simulink model "QPSK_ad9361_Solution"  (R2019a)
settings: Solver=ode23  StartTime=0.0  StopTime=inf  RelTol=1e-3  EnableMultiTasking=on
PreLoadFcn:
  | addpath('./filterwizard');
  | ad9361_preload(bdroot,'rx');
  | sdrqpsktx = qpsktx_init;
  | sdrqpskrx = qpskrx_init;
InitFcn:
  | sdrqpsktx = qpsktx_init;
  | sdrqpskrx = qpskrx_init;
undefined symbols (not defined in the file or in its folder): D, dBc, dBval, DCLeak_Matrix, dfilt, doppler, errordlg, Frame, fuzz_val, GainImb_Matrix, gcbh, IP2_Matrix, IP3_Matrix, magnitude, rcfiltgaincompat
libraries: simrfV2elements x23, dspmlti4 x10, simrfV2util1 x9, simulink x9, dsparch4 x8, fl_lib x7, dspmathops x5, dspobslib x4, simrfV2sources1 x3, simrfV2junction1 x3, commdigbbndpm3 x3, dspstat3 x3
(part 3 of 3)

== system QPSK_ad9361_Solution/ADI9361_tx1/DUC_Filters_TX/Hm3/Hm3 ==
  In : Inport
  Hm3 : dspmlti4/FIR Interpolation  FilterSource=Filter object  h=fir1(15,1/4)  L=3  FilterObject=ad9361_tx_pars.Hm3_tx  framing=Allow multirate processing  outputBufInitCond=0  roundingMode=Floor  overflowMode=off  firstCoeffDataTypeStr=Inherit: Same word length as input  firstCoeffMin=[]  firstCoeffMax=[]  firstCoeffLastDataTypeStr=Inherit: Same word length as input  outputDataTypeStr=Inherit: Same as accumulator  outputMin=[]  outputMax=[]  outputLastDataTypeStr=Inherit: Same as accumulator
      settings: SourceProductName=DSP System Toolbox
  Out : Outport
  wires:
  Hm3/1 -> Out/1
  In/1 -> Hm3/1

== system QPSK_ad9361_Solution/ADI9361_tx1/DUC_Filters_TX/Hm3/NoFilter ==
  In : Inport
  Out : Outport
  wires:
  In/1 -> Out/1

== system QPSK_ad9361_Solution/ADI9361_tx1/DUC_Filters_TX/Hm4/Hm4 ==
  In1 : Inport
  Hm4 : dspmlti4/FIR Interpolation  FilterSource=Filter object  h=fir1(15,1/4)  L=3  FilterObject=ad9361_tx_pars.Hm4_tx  framing=Allow multirate processing  outputBufInitCond=0  roundingMode=Floor  overflowMode=off  firstCoeffDataTypeStr=Inherit: Same word length as input  firstCoeffMin=[]  firstCoeffMax=[]  firstCoeffLastDataTypeStr=Inherit: Same word length as input  outputDataTypeStr=Inherit: Same as accumulator  outputMin=[]  outputMax=[]  outputLastDataTypeStr=Inherit: Same as accumulator
      settings: SourceProductName=DSP System Toolbox
  Out1 : Outport
  wires:
  Hm4/1 -> Out1/1
  In1/1 -> Hm4/1

== system QPSK_ad9361_Solution/ADI9361_tx1/DUC_Filters_TX/Hm4/NoFilter ==
  In1 : Inport
  Out1 : Outport
  wires:
  In1/1 -> Out1/1

== system QPSK_ad9361_Solution/ADI9361_tx1/RF_TX/Modulator/Combiner ==
  Gnd : fl_lib/Electrical/Electrical Elements/Electrical Reference
  Rl_I : simrfV2elements/R  classname=resistor  Resistance=50 Ohm  AddNoise=off
      settings: SourceProductName=RF Blockset  SourceProductBaseCode=RB
  Rl_Q : simrfV2elements/R  classname=resistor  Resistance=50 Ohm  AddNoise=off
      settings: SourceProductName=RF Blockset  SourceProductBaseCode=RB
  Rs : simrfV2elements/R  classname=resistor  Resistance=50 Ohm  AddNoise=off
      settings: SourceProductName=RF Blockset  SourceProductBaseCode=RB
  Signal Combiner : simrfV2elements/Signal Combiner  classname=signal_sum_mask  InternalGrounding=on
      settings: SourceProductName=RF Blockset  SourceProductBaseCode=RB
  In1 : PMIOPort  Side=Left
  In2 : PMIOPort  Port=2  Side=Left
  Out : PMIOPort  Port=3  Side=Right
  connections:
  Rs/RConn1 -- Signal Combiner/RConn1
  Rs/LConn1 -- Out/RConn1
  Rl_I/LConn1 -- In1/RConn1 -- Signal Combiner/LConn1
  Rl_Q/RConn1 -- In2/RConn1 -- Signal Combiner/LConn2
  Rl_I/RConn1 -- Rl_Q/LConn1 -- Gnd/LConn1

== system QPSK_ad9361_Solution/ADI9361_tx1/RF_TX/Modulator/GainImbalance = f(Attenuation,Imp) ==
  Attenuation : Inport
  1-D Lookup Table : Lookup_n-D  NumberOfTableDimensions=1  BreakpointsForDimension1="[    0    10    20    30    40    50    60    70    80]"  BreakpointsForDimension1FirstPoint=10  BreakpointsForDimension2FirstPoint=10  BreakpointsForDimension1Spacing=12  BreakpointsForDimension2Spacing=12  Table="[-55.5 -66.2 -53.5 -57.5 -44.5 -46.3 -54.2 -46.1 -34.3] / 20     %[dBc]"  InternalRulePriority=Speed  RndMeth=Simplest  InputSameDT=on
  Add : Sum
  Constant : Constant
  Control : Constant  Value=Imp
  Gain : Gain  Gain=20
  Gain1 : Gain  Gain=2
  Power : Math  Operator=10^u  SaturateOnIntegerOverflow=on
  Switch : Switch  Criteria=u2 ~= 0
  Zero : Constant  Value=0
  log10 : Math  Operator=log10  SaturateOnIntegerOverflow=on
  GainImbalance : Outport
  wires:
  log10/1 -> Gain/1
  Attenuation/1 -> 1-D Lookup Table/1
  Zero/1 -> Switch/3
  1-D Lookup Table/1 -> Power/1
  Gain/1 -> Switch/1
  Constant/1 -> Add/2
  Control/1 -> Switch/2
  Power/1 -> Gain1/1
  Gain1/1 -> Add/1
  Add/1 -> log10/1
  Switch/1 -> GainImbalance/1

== system QPSK_ad9361_Solution/ADI9361_tx1/RF_TX/Modulator/Noisy LO ==
  Constant : Constant  Value=sqrt(2)  VectorParams1D=off  SampleTime=1/Fs  FramePeriod=Frame/Fs
  Phase Noise : Subsystem  Description=|  mask{Level_dB=Level_dB, Freq=Freq, Fs=Fs, Npts=Npts, seed=seed, Verify=off}
      | User defined phase noise block.
      | Dick Benson, May 2007
      mask prompts: Level_dB "Noise Level Vector in dBc/Hz"; Freq "Frequency Vector in Hz"; Fs "Sampling Rate in Hz"; Npts "FIR Filter Kernel Length (power of 2)"; seed "Noise Gen. Seed"; Verify "Verify Noise Shape Attained"
      mask init:
      | noise_filt = phasenoise(Npts, Freq, Level_dB, Fs, Verify, gcb);
      mask Display: disp('Prototype\nPhase Noise\nBlock')
  Real-Imag to Complex : RealImagToComplex  Input=Real
  PLL Output : Outport
  wires:
  Constant/1 -> Real-Imag to Complex/1
  Real-Imag to Complex/1 -> Phase Noise/1(In1)
  Phase Noise/1(Out1) -> PLL Output/1

== system QPSK_ad9361_Solution/ADI9361_tx1/RF_TX/Modulator/R = f(Attenuation,Gain,Imp) ==
  Attenuation : Inport
  Add : Sum  Inputs=+-
  Constant : Constant  Value=50
  Constant2 : Constant  Value=1e21
  Control : Constant  Value=Imp
  Gain : Gain  Gain=50*50
  Lookup Table : Lookup_n-D  NumberOfTableDimensions=1  BreakpointsForDimension1="[  0  10  20  30  40  50   60   70   80]"  BreakpointsForDimension1FirstPoint=10  BreakpointsForDimension2FirstPoint=10  BreakpointsForDimension1Spacing=12  BreakpointsForDimension2Spacing=12  Table=-1*([-58 -52 -60 -71 -81 -82 -101 -102 -100] - Gain - 6)/10  InternalRulePriority=Speed  RndMeth=Simplest  InputSameDT=on
  Sqrt : Sqrt  SaturateOnIntegerOverflow=on
  Switch : Switch  Criteria=u2 ~= 0
  expon : Math  Operator=10^u  SaturateOnIntegerOverflow=on
  R : Outport
  wires:
  Constant/1 -> Add/2
  Lookup Table/1 -> expon/1
  Attenuation/1 -> Lookup Table/1
  Sqrt/1 -> Add/1
  Gain/1 -> Sqrt/1
  Control/1 -> Switch/2
  Switch/1 -> R/1
  Constant2/1 -> Switch/3
  Add/1 -> Switch/1
  expon/1 -> Gain/1

== system QPSK_ad9361_Solution/ADI9361_tx1/RF_TX/PA/OIP3 = f(Attenuation,OIP3v,Imp) ==
  Attenuation : Inport
  1-D Lookup Table : Lookup_n-D  NumberOfTableDimensions=1  BreakpointsForDimension1=[0 4 20 80]  BreakpointsForDimension1FirstPoint=10  BreakpointsForDimension2FirstPoint=10  BreakpointsForDimension1Spacing=12  BreakpointsForDimension2Spacing=12  Table=OIP3v  InternalRulePriority=Speed  RndMeth=Simplest  InputSameDT=on
  Constant2 : Constant  Value=500
  Control : Constant  Value=Imp
  Switch : Switch  Criteria=u2 ~= 0
  OIP3 : Outport
  wires:
  1-D Lookup Table/1 -> Switch/1
  Attenuation/1 -> 1-D Lookup Table/1
  Control/1 -> Switch/2
  Switch/1 -> OIP3/1
  Constant2/1 -> Switch/3

== system QPSK_ad9361_Solution/QPSK Receiver/Timing Recovery1/Modified Buffer/Modified Buffer ==
  In1 : Inport
  Enable : EnablePort
  Compare To Constant : simulink/Logic and Bit Operations/Compare To Constant  relop===  const=(bufSize-1)  OutDataTypeStr=boolean  ZeroCross=off
  Counter Limited : simulink/Sources/Counter Limited  uplimit=(bufSize-1)  tsamp=-1
  Delay Line : dspbuff3/Delay Line  siz=bufSize  ic=0  directfeed=on  enable_output=on  hold_output=off  OutputFrames=on
      settings: SourceProductName=DSP System Toolbox  SourceProductBaseCode=DS
  DataOut : Outport
  DataValid : Outport  Port=2
  wires:
  Compare To Constant/1 -> Delay Line/2, DataValid/1
  Delay Line/1 -> DataOut/1
  In1/1 -> Delay Line/1
  Counter Limited/1 -> Compare To Constant/1

== system QPSK_ad9361_Solution/QPSK Receiver/Timing Recovery1/Timing Recovery PLL/Loop Filter ==
  note: Proportional-Plus-Integrator Loop Filter,
      | Infinite DC Response to guarantee convergence
  e : Inport
  Digital Filter : dspobslib/Digital Filter  TypePopup=IIR (poles & zeros)  IIRFiltStruct=Direct form II transposed  AllPoleFiltStruct=Direct form  FIRFiltStruct=Direct form  CoeffSource=Specify via dialog  NumCoeffs=[1 0]  DenCoeffs=[1 -1]  BiQuadCoeffs=[1 0.3 0.4 1 0.1 0.2]  LatticeCoeffs=[0.2 0.4]  denIgnore=on  FiltPerSampPopup=One filter per frame  IC=0  ICnum=0  ICden=0  roundingMode=Floor  overflowMode=off  ScaleValues=1  scaleValueFracLength=14  stageInFracLength=15  stageOutFracLength=15  FilterSource=Specify via dialog  dfiltObjectName=dfilt.dffir([1 2 1])  InputProcessing=Columns as channels (frame based)
      settings: SourceProductName=DSP System Toolbox  SourceProductBaseCode=DS
  K1 : Gain  Gain=K1
  K2 : Gain  Gain=K2
  Sum2 : Sum  SaturateOnIntegerOverflow=on  InputSameDT=on  OutDataTypeStr=Inherit: Same as first input
  v : Outport
  wires:
  K2/1 -> Digital Filter/1
  Digital Filter/1 -> Sum2/2
  Sum2/1 -> v/1
  e/1 -> K2/1, K1/1
  K1/1 -> Sum2/1

== system QPSK_ad9361_Solution/ADI9361_rx1/RF_RX/RF Receiver/Demodulator/R = f(gain, DCleak) ==
  gain : Inport
  DCleak : Inport  Port=2
  Add : Sum  Inputs=--+-+
  Add1 : Sum  Inputs=+-
  Constant1 : Constant  Value=20
  Constant2 : Constant  Value=27
  Constant3 : Constant  Value=3
  Constant4 : Constant  Value=25
  Gain1 : Gain  Gain=(-1)/20
  Gain2 : Gain  Gain=25
  expon3 : Math  Operator=10^u  SaturateOnIntegerOverflow=on
  R : Outport
  wires:
  Add1/1 -> R/1
  Constant4/1 -> Add1/2
  Gain2/1 -> Add1/1
  Gain1/1 -> expon3/1
  Constant2/1 -> Add/4
  Constant1/1 -> Add/3
  Constant3/1 -> Add/2
  DCleak/1 -> Add/5
  Add/1 -> Gain1/1
  gain/1 -> Add/1
  expon3/1 -> Gain2/1

== system QPSK_ad9361_Solution/ADI9361_rx1/RF_RX/RF Receiver/Demodulator/y = f(gain, gainImbalance) ==
  gain : Inport
  gainImbalance : Inport  Port=2
  Add2 : Sum
  Constant2 : Constant  Value=2
  Gain4 : Gain  Gain=1/20
  Gain5 : Gain  Gain=1/20
  Gain6 : Gain  Gain=20
  Times1 : Product  Inputs=***
  expon2 : Math  Operator=10^u  SaturateOnIntegerOverflow=on
  expon3 : Math  Operator=10^u  SaturateOnIntegerOverflow=on
  log1 : Math  Operator=log10  SaturateOnIntegerOverflow=on
  y : Outport
  wires:
  expon2/1 -> Times1/2
  Gain5/1 -> expon3/1
  Times1/1 -> Add2/2
  Gain4/1 -> expon2/1
  Add2/1 -> log1/1
  log1/1 -> Gain6/1
  gain/1 -> Gain5/1
  expon3/1 -> Times1/1, Add2/1
  gainImbalance/1 -> Gain4/1
  Constant2/1 -> Times1/3
  Gain6/1 -> y/1

== system QPSK_ad9361_Solution/ADI9361_rx1/RF_RX/RF Receiver/External LNA/Invert Control ==
  In : Inport
  Data Type Conversion : DataTypeConversion  OutDataTypeStr=boolean
  Data Type Conversion1 : DataTypeConversion  OutDataTypeStr=double
  Logical Operator : Logic  Operator=NOT  AllPortsSameDT=off  OutDataTypeStr=boolean
  Out : Outport
  wires:
  In/1 -> Data Type Conversion/1
  Logical Operator/1 -> Data Type Conversion1/1
  Data Type Conversion/1 -> Logical Operator/1
  Data Type Conversion1/1 -> Out/1

== system QPSK_ad9361_Solution/ADI9361_rx1/RF_RX/RF Receiver/RF Non Idealities/DetectChange ==
  In1 : Inport
  In2 : Inport  Port=2
  In3 : Inport  Port=3
  In4 : Inport  Port=4
  Detect Change{,1..4} (5 alike) : simulink/Logic and Bit Operations/Detect Change  vinit=0  InputProcessing=Inherited  OutDataTypeStr=boolean
  Logical Operator : Logic  Operator=OR  Inputs=5  AllPortsSameDT=off  OutDataTypeStr=boolean
  Step : Step  Time=2*Tstep  SampleTime=Tstep  VectorParams1D=off  ZeroCross=off
  Trigger : Outport
  wires:
  Detect Change/1 -> Logical Operator/4
  Detect Change1/1 -> Logical Operator/3
  Detect Change2/1 -> Logical Operator/2
  In4/1 -> Detect Change3/1
  In2/1 -> Detect Change1/1
  In3/1 -> Detect Change2/1
  Detect Change3/1 -> Logical Operator/1
  In1/1 -> Detect Change/1
  Logical Operator/1 -> Trigger/1
  Detect Change4/1 -> Logical Operator/5
  Step/1 -> Detect Change4/1

== system QPSK_ad9361_Solution/ADI9361_rx1/RF_RX/RF Receiver/RF Non Idealities/RF Non Idealities ==
  LNA : Inport
  Demod : Inport  Port=2
  TIA : Inport  Port=3
  LPF : Inport  Port=4
  Trigger : TriggerPort  VariantControl=Variant  PortDimensions=1
  RF NonIdealities : MATLAB Function  TreatAsAtomicUnit=on
      mask init:
      | load ADI9361Tables;
  DCLeakage : Outport
  GainImbalance : Outport  Port=2
  IP2 : Outport  Port=3
  IP3 : Outport  Port=4
  wires:
  RF NonIdealities/1(Leak) -> DCLeakage/1
  RF NonIdealities/2(GainImb) -> GainImbalance/1
  RF NonIdealities/3(IP2) -> IP2/1
  RF NonIdealities/4(IP3) -> IP3/1
  LNA/1 -> RF NonIdealities/1(LNA)
  LPF/1 -> RF NonIdealities/4(LPF)
  Demod/1 -> RF NonIdealities/2(Demod)
  TIA/1 -> RF NonIdealities/3(TIA)

== system QPSK_ad9361_Solution/ADI9361_tx1/RF_TX/Modulator/Noisy LO/Phase Noise ==
  In1 : Inport
  Digital Filter : dspobslib/Digital Filter  TypePopup=FIR (all zeros)  IIRFiltStruct=Direct form II transposed  AllPoleFiltStruct=Direct form  FIRFiltStruct=Direct form  CoeffSource=Specify via dialog  NumCoeffs=noise_filt*sqrt(Fs)  DenCoeffs=den  BiQuadCoeffs=[1 0.3 0.4 1 0.1 0.2]  LatticeCoeffs=[0.2 0.4]  denIgnore=on  FiltPerSampPopup=One filter per frame  IC=0  ICnum=0  ICden=0  roundingMode=Floor  overflowMode=off  ScaleValues=1  scaleValueFracLength=14  stageInFracLength=15  stageOutFracLength=15  FilterSource=Specify via dialog  dfiltObjectName=dfilt.dffir([1 2 1])  InputProcessing=Inherited (this choice will be removed - see release notes)
      settings: SourceProductName=DSP System Toolbox  SourceProductBaseCode=DS
  Magnitude-Angle to Complex : MagnitudeAngleToComplex  Input=Angle  ConstantPart=1
  Noise Source : Subsystem
      mask Display: disp('Noise Source')
  Product : Product  SaturateOnIntegerOverflow=on  InputSameDT=on  OutDataTypeStr=Inherit: Same as first input
  Out1 : Outport
  wires:
  In1/1 -> Product/1, Noise Source/1(In1)
  Product/1 -> Out1/1
  Digital Filter/1 -> Magnitude-Angle to Complex/1
  Noise Source/1(Out1) -> Digital Filter/1
  Magnitude-Angle to Complex/1 -> Product/2

== system QPSK_ad9361_Solution/ADI9361_tx1/RF_TX/Modulator/Noisy LO/Phase Noise/Noise Source ==
  In1 : Inport
  AWGN Channel : commchan3/AWGN Channel  InputProcessing=Inherited (this choice will be removed - see release notes)  seed=12598763  noiseMode=Variance from mask  EbNodB=10  EsNodB=10  SNRdB=0  bitsPerSym=1  Ps=1  Tsym=1  variance=2
      settings: SourceProductName=Communications Toolbox
  Complex to Real-Imag : ComplexToRealImag  Output=Real
  Sum : Sum  Inputs=-+|  SaturateOnIntegerOverflow=on  InputSameDT=on  OutDataTypeStr=Inherit: Same as first input
  Out1 : Outport
  wires:
  Sum/1 -> Complex to Real-Imag/1
  AWGN Channel/1 -> Sum/2
  In1/1 -> AWGN Channel/1, Sum/1
  Complex to Real-Imag/1 -> Out1/1

== matlab function QPSK_ad9361_Solution/QPSK TX/Bit Generation/Message Source/Message Generator ==
  data: msg output
function msg = genMsg
%#codegen
persistent msgStrSet count;
if isempty(msgStrSet)
    count = 0;
    msgStrSet = ['Hello world 000';...
              'Hello world 001';...
              'Hello world 002';...
              'Hello world 003';...
              'Hello world 004';...
              'Hello world 005';...
              'Hello world 006';...
              'Hello world 007';...
              'Hello world 008';...
              'Hello world 009';...
              'Hello world 010';...
              'Hello world 011';...
              'Hello world 012';...
              'Hello world 013';...
              'Hello world 014';...
              'Hello world 015';...
              'Hello world 016';...
              'Hello world 017';...
              'Hello world 018';...
              'Hello world 019';...
              'Hello world 020';...
              'Hello world 021';...
              'Hello world 022';...
              'Hello world 023';...
              'Hello world 024';...
              'Hello world 025';...
              'Hello world 026';...
              'Hello world 027';...
              'Hello world 028';...
              'Hello world 029';...
              'Hello world 030';...
              'Hello world 031';...
              'Hello world 032';...
              'Hello world 033';...
              'Hello world 034';...
              'Hello world 035';...
              'Hello world 036';...
              'Hello world 037';...
              'Hello world 038';...
              'Hello world 039';...
              'Hello world 040';...
              'Hello world 041';...
              'Hello world 042';...
              'Hello world 043';...
              'Hello world 044';...
              'Hello world 045';...
              'Hello world 046';...
              'Hello world 047';...
              'Hello world 048';...
              'Hello world 049';...
              'Hello world 050';...
              'Hello world 051';...
              'Hello world 052';...
              'Hello world 053';...
              'Hello world 054';...
              'Hello world 055';...
              'Hello world 056';...
              'Hello world 057';...
              'Hello world 058';...
              'Hello world 059';...
              'Hello world 060';...
              'Hello world 061';...
              'Hello world 062';...
              'Hello world 063';...
              'Hello world 064';...
              'Hello world 065';...
              'Hello world 066';...
              'Hello world 067';...
              'Hello world 068';...
              'Hello world 069';...
              'Hello world 070';...
              'Hello world 071';...
              'Hello world 072';...
              'Hello world 073';...
              'Hello world 074';...
              'Hello world 075';...
              'Hello world 076';...
              'Hello world 077';...
              'Hello world 078';...
              'Hello world 079';...
              'Hello world 080';...
              'Hello world 081';...
              'Hello world 082';...
              'Hello world 083';...
              'Hello world 084';...
              'Hello world 085';...
              'Hello world 086';...
              'Hello world 087';...
              'Hello world 088';...
              'Hello world 089';...
              'Hello world 090';...
              'Hello world 091';...
              'Hello world 092';...
              'Hello world 093';...
              'Hello world 094';...
              'Hello world 095';...
              'Hello world 096';...
              'Hello world 097';...
              'Hello world 098';...
              'Hello world 099'];              
end
msgStr = msgStrSet(count+1,:);
msgBin = de2bi(int8(msgStr),7,'left-msb');
msg = reshape(double(msgBin).',105,1);
count = mod(count+1,100);

== stateflow chart QPSK_ad9361_Solution/ADI9361_rx1/AGC ==
  settings: executeAtInitialization=1
  state InitialState
    entry: gain_index=76;
  state SLOW
  state MGC
  state DECREASE_GAIN_AGC_Inner
    entry:
    gain_index = max(gain_index-AGC_G_dec_slow,0);
  state DoNothing
  state CHANGE_GAIN
    entry:
    gain_index = ManualGainIndex;
  state INCREASE_GAIN_Inner
    entry:
    gain_index = min(gain_index+AGC_G_inc_slow,76);
  state DECREASE_GAIN_AGC_Outer
    entry:
    gain_index = max(gain_index-AGC_G_dec_fast,0);
  state INCREASE_GAIN_Outer
    entry:
    gain_index = min(gain_index+AGC_G_inc_fast,76);
  state DECREASE_GAIN_ADC
    entry:
    gain_index = max(gain_index-ADC_G_dec_fast,0);
  state DECREASE_GAIN_LMT
    entry:
    gain_index = max(gain_index-LMT_G_dec_fast,0);
  (default) -> InitialState
  InitialState -> (junction 14) : after(T*1e-6,sec)
  (junction 14) -> MGC [order 2] : [mode==1]/{gain_index = ManualGainIndex;}
  (junction 14) -> SLOW [order 1] : [mode==0]
  MGC -> (junction 14) [order 2] : [mode==0]
  SLOW -> (junction 14) [order 1] : [mode==1]
  CHANGE_GAIN -> MGC : after(1e-9,sec)
  MGC -> CHANGE_GAIN [order 1] : [hasChanged(ManualGainIndex)]
  DECREASE_GAIN_LMT -> SLOW : after(C*1e-6,sec)
  SLOW -> DECREASE_GAIN_LMT [order 2] : at(N_LMT_H, LMT_H)
  DECREASE_GAIN_ADC -> SLOW : after(C*1e-6,sec)
  SLOW -> DECREASE_GAIN_ADC [order 3] : at(N_ADC_H, ADC_H)
  DECREASE_GAIN_AGC_Outer -> SLOW : after(C*1e-6,sec)
  SLOW -> DECREASE_GAIN_AGC_Outer [order 4] : at(1, POW_H_outer)
  DECREASE_GAIN_AGC_Inner -> SLOW : after(C*1e-6,sec)
  SLOW -> DECREASE_GAIN_AGC_Inner [order 5] : at(1, POW_H_inner)
  INCREASE_GAIN_Outer -> SLOW : after(C*1e-6,sec)
  SLOW -> INCREASE_GAIN_Outer [order 6] : at(1, POW_L_outer)
  INCREASE_GAIN_Inner -> SLOW : after(C*1e-6,sec)
  SLOW -> INCREASE_GAIN_Inner [order 7] : at(1, POW_L_inner)
  DoNothing -> SLOW
  SLOW -> DoNothing [order 8] : at(N_LMT_L, LMT_L)
  SLOW -> DoNothing [order 9] : at(N_ADC_L,ADC_L)
  data: mode input; N_LMT_H parameter double; N_LMT_L parameter double; N_ADC_H parameter double; N_ADC_L parameter double; gain_index output double; C parameter; ManualGainIndex input double; ADC_G_dec_fast parameter; AGC_G_inc_fast parameter; AGC_G_inc_slow parameter; LMT_G_dec_fast parameter; T parameter; AGC_G_dec_fast parameter; AGC_G_dec_slow parameter
  events: POW_L_outer input RISING_EDGE_EVENT; POW_L_inner input RISING_EDGE_EVENT; POW_H_inner input RISING_EDGE_EVENT; POW_H_outer input RISING_EDGE_EVENT; ADC_H input RISING_EDGE_EVENT; ADC_L input RISING_EDGE_EVENT; LMT_L input RISING_EDGE_EVENT; LMT_H input RISING_EDGE_EVENT; event input RISING_EDGE_EVENT

== matlab function QPSK_ad9361_Solution/ADI9361_rx1/RF_RX/RF Receiver/RF Non Idealities/RF Non Idealities/RF NonIdealities ==
  data: LNA input; Leak output; Demod input; TIA input; LPF input; GainImb output; IP2 output; IP3 output; DCLeak_Matrix parameter; GainImb_Matrix parameter; IP3_Matrix parameter; IP2_Matrix parameter
function [Leak, GainImb, IP2, IP3] =                                    ...
    nonIdealsRF(LNA, Demod, TIA, LPF, DCLeak_Matrix, GainImb_Matrix,    ...
    IP3_Matrix, IP2_Matrix)
%#codegen
coder.extrinsic('griddatan','warning');
IP2 = 200;
IP3 = 200;
Leak = -200;
GainImb = -200;
Leak(:) = griddatan(DCLeak_Matrix(:,1:4), DCLeak_Matrix(:,5),           ...
    [LNA, Demod, TIA, LPF]);
GainImb(:) = griddatan(GainImb_Matrix(:,1:4), GainImb_Matrix(:,5),      ...
    [LNA, Demod, TIA, LPF]);
IP2(:) = griddatan(IP2_Matrix(:,1:4), IP2_Matrix(:,5),[LNA,Demod,TIA,LPF]);
IP3(:) = griddatan(IP3_Matrix(:,1:4), IP3_Matrix(:,5),[LNA,Demod,TIA,LPF]);

if isnan(IP2)
    IP2(:) = griddatan(IP2_Matrix(:,1:4), IP2_Matrix(:,5),              ...
        [LNA, Demod, TIA, LPF],'nearest');
    % Warning('Failed interpolation on IP2');
end
if isnan(IP3)
    IP3(:) = griddatan(IP3_Matrix(:,1:4), IP3_Matrix(:,5),              ...
        [LNA, Demod, TIA, LPF],'nearest');
    % Warning('Failed interpolation on IP3');
end
if isnan(Leak)
    Leak(:) = griddatan(DCLeak_Matrix(:,1:4), DCLeak_Matrix(:,5),       ...
        [LNA, Demod, TIA, LPF],'nearest');
    % Warning('Failed interpolation on DC leakage');
end
if isnan(GainImb)
    GainImb(:) = griddatan(GainImb_Matrix(:,1:4), GainImb_Matrix(:,5),  ...
        [LNA, Demod, TIA, LPF],'nearest');
    % Warning('Failed interpolation on Gain Imbalance');
end

IP2 = 2*(IP2+LNA);

== matlab function QPSK_ad9361_Solution/QPSK Receiver/Coarse Frequency Compensation1/Find Frequency Offset/Find Frequency Offset ==
  data: N input; FreqOffset output; Tf input; FFTSig input; M parameter
function FreqOffset = findfreqoffset(N,Tf,FFTSig,M) %#codegen
%  Estimate frequency offset.
%  findfreqoffset(N,Tf,fvec,params) returns the estimated frequency offset
%  given time-domain frame length N, sample time vector Tf containing
%  [frameTime,offsetTime], complex FFT vector FFTsig, and modulation
%  order M.

% Find index of max magnitude, convert to offset symmetric about zero.
% Return a negative integer offset to be interpreted as a compensation.
[~,maxIdx] = max(FFTSig);
FFTSize = size(FFTSig,1);
if maxIdx > FFTSize/2
    OffsetIdx = FFTSize+1-maxIdx;
else
    OffsetIdx = 1-maxIdx;
end
% Map offset index to a frequency value.
% Compute offset using modulation alphabet size params.M.
Ts = Tf(1)/N; % Sample time
delta_f = 1/(Ts*FFTSize); % Frequency resolution of FFT
FreqOffset = OffsetIdx * delta_f / M;

== matlab function QPSK_ad9361_Solution/QPSK Receiver/Data Decoding1/Align Data ==
  data: Delay input; RxData input; Data output
function Data  = aligndata(Delay, RxData)
% Extract data from the buffered RxData, using the delay to find the frame 
% start
%
% Input:
% Delay - Index of frame start
% RxData - Buffered symbol-spaced data
% Output:
% Data - Data with the Barker code at frame start
%#codegen
Data = RxData(Delay+1:Delay+length(RxData)/2);

== matlab function QPSK_ad9361_Solution/QPSK Receiver/Data Decoding1/BitsToDecimal ==
  data: u input
function BitsToASCII(u)
% Convert bits to ASCII message.

coder.extrinsic('disp')

% Convert binary-valued column vector to 7-bit decimal values.
w = [64 32 16 8 4 2 1]; % binary digit weighting
Nbits = numel(u);
Ny = Nbits/7;
y = zeros(1,Ny);
for i = 0:Ny-1
    y(i+1) = w*u(7*i+(1:7));
end

% Display ASCII message to command window
disp(char(y));

== matlab function QPSK_ad9361_Solution/QPSK Receiver/Data Decoding1/Phase Offset Estimator/Phase Offset Detection ==
  data: In input; Out output
function Out = phasedecision(In)
% Map the estimated phase to one of -pi, -pi/2, 0, pi/2,  
%#codegen
% Out = round(In.*2./pi)./2.*pi;
% The above processing is equivalent to the following processing using
% if/else statements
%
% if In<pi/4 && In>-pi/4
%     Out = 0;
% elseif In>=pi/4 && In<pi*3/4
%     Out = pi/2;
% elseif In>=pi*3/4 || In<=-pi*3/4
%     Out = -pi;
% else
%     Out = -pi/2;
% end

if In<pi/4 && In>=-pi/4
    Out = 0;
elseif In>=pi/4 && In<pi*3/4
    Out = pi/2;
elseif In>=pi*3/4 || In<-pi*3/4
    Out = -pi;
else
    Out = -pi/2;
end

== matlab function QPSK_ad9361_Solution/QPSK Receiver/Fine Frequency Compensation1/PED ==
  data: In input; e output
function e = PED(In)
% Implementation of Maximum Likelihood Phase Error Detector listed in
% Chapter 7.2.2 of "Digital Communications - A Discrete-Time Approach" by
% Michael Rice. This employs a decision directed method.
% 
% Input: 
%   In - Input samples, oversampled by two
% Output:
%   e - Phase error, de
%#codegen

e = sign(real(In)).*imag(In) - sign(imag(In)).*real(In);

== matlab function QPSK_ad9361_Solution/QPSK Receiver/Timing Recovery1/Timing Recovery PLL/Interpolation Filter ==
  data: In input; Out output; mu input
function Out = interp_filter(In, mu)
% Prabolic piecewise polynomial interpolator, Farrow Interpolator with 
% alpha = 1/2, see Figure 8.4.16 of "Digital Communications - A 
% Discrete-Time Approach" by Michael Rice.
% Input:
%   In - Input samples, oversampled by two
%   mu - Difference between actual sampling instant and the optimal instant,
%        between zero and one
% Output:
%   Out - Interpolation output
%#codegen
persistent delay1 delay2 delay3; % Input delayed by 1, 2 and 3 samples
if isempty(delay1)
    [delay1, delay2, delay3] = deal(complex(0,0));
end

K = -0.5;

Out = delay2 + mu.*(K.*(In+delay2+delay3)+(1-K).*delay1)...
      + K.*(delay1+delay2-In-delay3).*mu.^2;
  
% Update delay buffers
delay3 = delay2;
delay2 = delay1;
delay1 = In;

== matlab function QPSK_ad9361_Solution/QPSK Receiver/Timing Recovery1/Timing Recovery PLL/NCO Control ==
  data: Delta input; Underflow output; mu output; sdrqpskrx parameter
function [Underflow, mu] = NCO_ctrl(Delta, sdrqpskrx)
% Implementation of modulo-1 counter for interpolation control listed in
% Figure 8.4.19 of "Digital Communications - A Discrete-Time Approach"
% by Michael Rice. See design details in Chapter 8.4.3 of the same book.
% 
% Input:
%   Delta - Loop filter output. If loop is in lock, delta would be small
%   qpsktxrx - Simulation parameter structure
% Output:
%   Underflow - Indicator of counter underflow. This is the strobe signal
%   for downstream processing
%   mu - Difference between actual sampling instant and the optimal instant,
%        between zero and one
%#codegen

% delay1 - Counter value delayed by 1 sample
% Regtemp - The estimated timing error normalized by half QPSK symbols
persistent delay1 Regtemp;  
if isempty(delay1)
    [delay1, Regtemp] = deal(0);
end
Upsampling = sdrqpskrx.Upsampling;
Downsampling = sdrqpskrx.Downsampling;
oversampling = Upsampling/Downsampling;

counter = mod(delay1,1)-Delta-1/oversampling; % decrementing counter
if counter < 0
    Underflow = 1;
    Regtemp = mod(delay1,1)/(Delta+1/oversampling);
else
    Underflow = 0;
end

mu = Regtemp;

% Update delay buffer
delay1 = mod(delay1,1)-Delta-1/oversampling;

== matlab function QPSK_ad9361_Solution/QPSK Receiver/Timing Recovery1/Timing Recovery PLL/Timing Error Detector ==
  data: In input; e output; strobe input
function e = TED(In, strobe)
% Zero-Crossing Timing Error Detector. See "Zero-Crossing Timing Error
% Detector" section in Chapter 8.4.1 of "Digital Communications - A
% Discrete-Time Approach" by Michael Rice. For bit stuffing/stripping
% details, see page 490-494 of the same book.
%
% Input: 
%   In - Input samples, interpolation result
%   strobe - Signal to enable timing error calculation
% Output:
%   e - Timing error
%#codegen
persistent delay1 delay2 delayStrobe; % Input delayed by one and 2 samples, and
% Enable signal delayed by one sample
if isempty(delay1)
    [delay1, delay2] = deal(complex(0,0));
    delayStrobe = 0;
end

if strobe==1 && delayStrobe~=strobe
    e = real(delay1) * (sign(real(delay2)) - sign(real(In))) + ...
        imag(delay1) * (sign(imag(delay2)) - sign(imag(In)));
else
    e = 0;
end

if delayStrobe~=strobe
    % Shift contents in delay register
    delay2 = delay1;
    delay1 = In;
elseif strobe==1
    % Two consecutive high strobes
    delay2 = 0; % Stuff missing sample
    delay1 = In; 
end
% If both current and previous enable signals are 0, skip current sample
% and keep the delayed signals unchanged. (Bit stripping)
delayStrobe = strobe;
